simulink model "TrafficLight_module"  (R2024b)
settings: Solver=VariableStepAuto  StartTime=0.0  StopTime=inf  RelTol=1e-3
settings Model: Creator=sudee  LastModifiedBy=91636

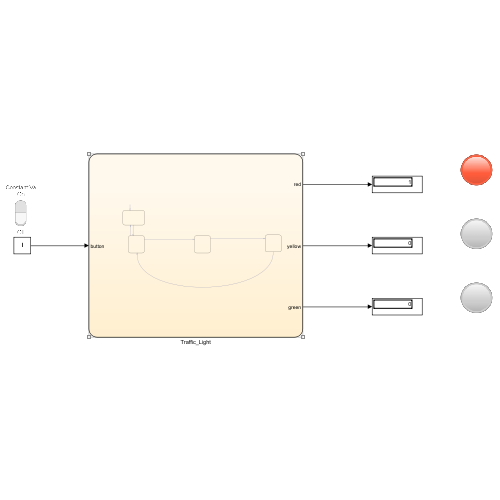
[thumbnail: Simulink's stored preview of the top-level diagram]
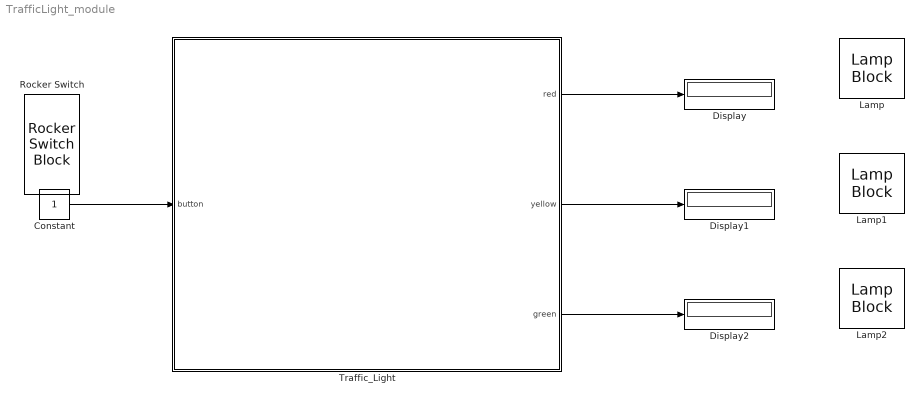
== system TrafficLight_module ==
  Constant : Constant
  Display : Display
  Display1 : Display
  Display2 : Display
  Lamp : LampBlock  LabelPosition=Hide
  Lamp1 : LampBlock  LabelPosition=Hide
  Lamp2 : LampBlock  LabelPosition=Hide
  Rocker Switch : RockerSwitchBlock
      settings: Values={{'Off', 'On'}, [0 1]}
  Traffic_Light : Stateflow chart  TreatAsAtomicUnit=on
  wires:
  Traffic_Light/3(green) -> Display2/1
  Traffic_Light/2(yellow) -> Display1/1
  Traffic_Light/1(red) -> Display/1
  Constant/1 -> Traffic_Light/1(button)

== stateflow chart TrafficLight_module/Traffic_Light ==
  state On_off
    entry:
    green=0;
    yellow=0;
    red=0;
  state Go
    entry:
    yellow=0;
    during:
    green=1;
  state Stop
    entry:
    green=0;
    during:
    red=1;
  state Be_Ready
    entry:
    red=0;
    during:
    yellow=1;
  (default) -> On_off
  Stop -> On_off [order 2] : [button==0]
  On_off -> Stop : [button==1]
  Be_Ready -> Go : [after(5, sec)]
  Stop -> Be_Ready [order 1] : [after(5, sec)]
  Go -> Stop : [after(5, sec)]
  data: red output; yellow output; green output; button input
